simulink model "ros_with_simulink"  (Simulink 8.7)
settings: Solver=VariableStepAuto  StartTime=0.0  StopTime=100  RelTol=1e-3
PreLoadFcn:
  | load center.mat;
  | Xref_ = center(1,:) * 43;
  | Yref_ = center(2,:) * 43;
  | 
  | Xref_ = Xref_ - Xref_(1);
  | Yref_ = Yref_ - Yref_(1);
  | 
  | Xref_ = Xref_(1,1:end);
  | Yref_ = Yref_(1,1:end);
  | 
  | N = size(Xref_);
  | N = N(2);
  | % Yref 世界坐标系 → frenet坐标系
  | [s_,rx,ry,rs,ryaw,rk] = convert_s(Xref_,Yref_);
  | rpath = [rx,ry,rs,ryaw,rk];
  | 
  | global v_acutal;
  | global deltaf_actual;
  | deltaf_actual = 0;
  | v_actual = 0;
undefined symbols (not defined in the file): Orientation, Position
libraries: robotlib x3, Solver_SF x1, simulink x1
settings Model: Creator=HY  LastModifiedBy=HY
settings DataIOCC: LimitDataPoints=off  SaveFormat=Dataset
settings DebuggingCC: UnderspecifiedInitializationDetection=Simplified  MergeDetectMultiDrivingBlocksExec=error
settings HardwareCC: ProdBitPerPointer=64  ProdLargestAtomicFloat=Float  ProdIntDivRoundTo=Zero  ProdEndianess=LittleEndian  ProdWordSize=64  ProdHWDeviceType=Intel->x86-64 (Windows64)
settings ModelReferenceCC: PropagateSignalLabelsOutOfModel=on
settings ConfigComp: CovModelRefEnable=off

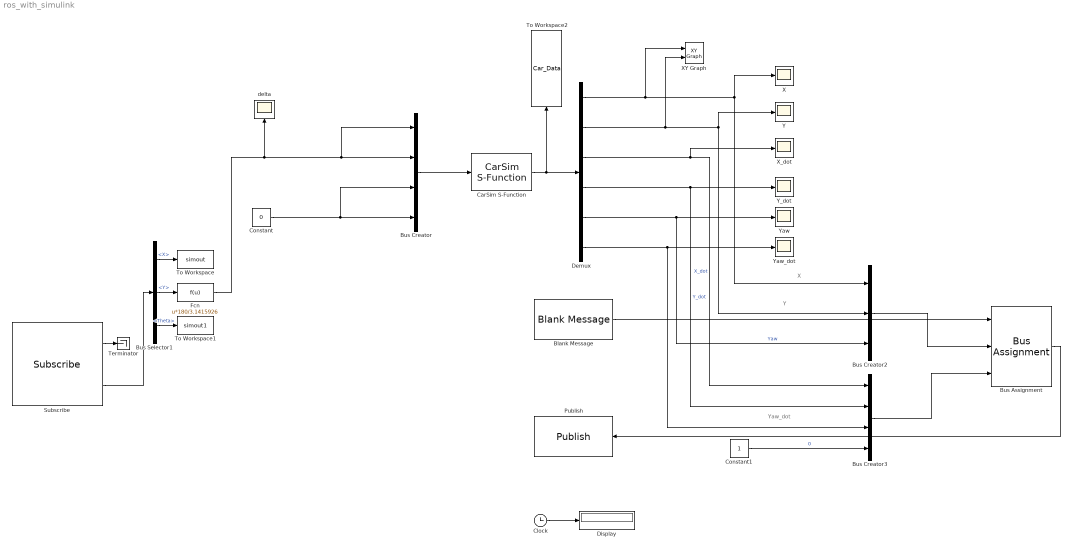
== system ros_with_simulink ==
  note: Yaw_dot
  note: Y
  note: X
  Blank Message : robotlib/Blank Message  SourceLibraryInfo=This block requires Robotics System Toolbox  messageType=geometry_msgs/Pose  SampleTime=-1
  Bus Assignment : BusAssignment  AssignedSignals=Position,Orientation
  Bus Creator : BusCreator  Inputs=4
  Bus Creator2 : BusCreator  Inputs=3
  Bus Creator3 : BusCreator  Inputs=4
  Bus Selector1 : BusSelector  OutputSignals=X,Y,Theta
  CarSim S-Function : Solver_SF/CarSim S-Function  Priority=1  VehicleCode=i_i  SIMFILE=simfile
  Clock : Clock
  Constant : Constant  Value=0
  Constant1 : Constant
  Demux : Demux  Outputs=6
  Display : Display
  Fcn : Fcn  Expr=u*180/3.1415926
  Publish : robotlib/Publish  SourceLibraryInfo=This block requires Robotics System Toolbox  topicSource=Specify your own  topic=/simulink_pose  messageType=geometry_msgs/Pose  messageQueueLength=1
  Subscribe : robotlib/Subscribe  SourceLibraryInfo=This block requires Robotics System Toolbox  topicSource=Specify your own  topic=/control  messageType=geometry_msgs/Pose2D  sampleTime=-1  messageQueueLength=1
  Terminator : Terminator
  To Workspace : ToWorkspace  VariableName=simout  SaveFormat=Timeseries  SampleTime=-1
  To Workspace1 : ToWorkspace  VariableName=simout1  SaveFormat=Timeseries  SampleTime=-1
  To Workspace2 : ToWorkspace  VariableName=Car_Data  SaveFormat=Timeseries  SampleTime=-1
  X : Scope
  XY Graph : simulink/Sinks/XY Graph  xmin=-20  xmax=150  ymin=-150  ymax=20  st=-1
  X_dot : Scope
  Y : Scope
  Y_dot : Scope
  Yaw : Scope
  Yaw_dot : Scope
  delta : Scope
  wires:
  Subscribe/2 -> Bus Selector1/1
  Bus Assignment/1 -> Publish/1
  CarSim S-Function/1 -> Demux/1, To Workspace2/1
  Clock/1 -> Display/1
  Subscribe/1 -> Terminator/1
  Blank Message/1 -> Bus Assignment/1
  Demux/1 -> XY Graph/1, Bus Creator2/1, X/1
  Demux/2 -> XY Graph/2, Bus Creator2/2, Y/1
  Demux/3 -> Bus Creator3/1, X_dot/1  "X_dot"
  Demux/5 -> Bus Creator2/3, Yaw/1  "Yaw"
  Demux/6 -> Bus Creator3/3, Yaw_dot/1
  Constant/1 -> Bus Creator/3, Bus Creator/4
  Bus Creator/1 -> CarSim S-Function/1
  Bus Selector1/2 -> Fcn/1  "<Y>"
  Fcn/1 -> delta/1, Bus Creator/1, Bus Creator/2
  Bus Selector1/1 -> To Workspace/1  "<X>"
  Bus Selector1/3 -> To Workspace1/1  "<Theta>"
  Demux/4 -> Bus Creator3/2, Y_dot/1  "Y_dot"
  Constant1/1 -> Bus Creator3/4  "0"
  Bus Creator2/1 -> Bus Assignment/2
  Bus Creator3/1 -> Bus Assignment/3
